simulink model "singlependulum_2"  (R2025a)
settings: Solver=ode15s  StartTime=0.0  StopTime=20  RelTol=1e-3
libraries: fl_lib x32, ee_lib x9, nesl_utility x5
settings Model: Creator=yang  LastModifiedBy=yang

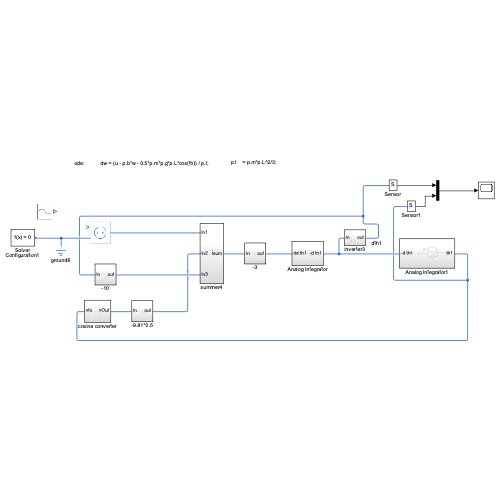
[thumbnail: Simulink's stored preview of the top-level diagram]
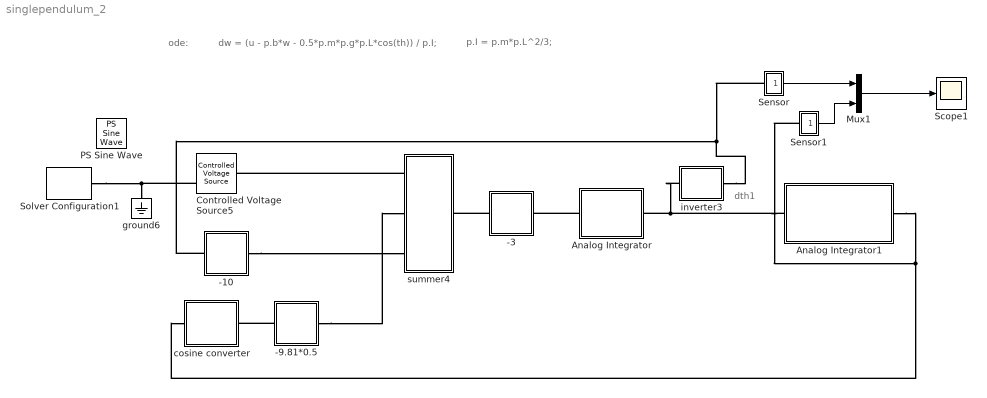
== system singlependulum_2 ==
  note: dth1
  note: ode:
  note: p.I = p.m*p.L^2/3;
  note: dw = (u - p.b*w - 0.5*p.m*p.g*p.L*cos(th)) / p.I;
  -10 : Subsystem
  -3 : Subsystem
  -9.81*0.5 : Subsystem
  Analog Integrator : Subsystem
  Analog Integrator1 : Subsystem
  Controlled Voltage Source5 : fl_lib/Electrical/Electrical Sources/Controlled Voltage Source
  Mux1 : Mux  Inputs=2
  PS Sine Wave : fl_lib/Physical Signals/Sources/PS Sine Wave  amplitude=5  bias=0  frequency_spec=foundation.enum.frequencySpec.angular  frequency_SI=5 Hz  frequency_angular=5 rad/s  phase=0 rad
      settings: InternalSimscapePortConfiguration="{\"Bottom\":[],\"Left\":[],\"Right\":[{\"id\":\"O\",\"label\":\"\",\"type\":\"output\"}],\"Top\":[]}"
  Scope1 : Scope
      settings: ActiveDisplayYMinimum=-2.4953450828768631  ActiveDisplayYMaximum=1.4302884628239119
  Sensor : Subsystem
      mask Display: disp('S')
  Sensor1 : Subsystem
      mask Display: disp('S')
  Solver Configuration1 : nesl_utility/Solver Configuration  PhysicalDomain=network_engine_domain  SubClassName=solver  LeftPortType=input  RightPortType=generic  Tones=[]  Harmonics=[]  SimulateNoise=off  Profile=off  UseLocalSampling=off  EnableSwitchedLinearOptims=on  FrequencyDomain=off  UseCCode=off  RelTol=0.001  AbsTol=1e-06  MinStep=1e-09  ToWorkspace=off  RevertToSquareIcSolve=off  NumHomotopyIterations=100  PhasorMode=off  PhasorModeNumHarmonics=1  ConsistencySolver=NEWTON_XTOL_AFTER_FTOL  IndexReductionMethod=DerivativeReplacement  DoDC=off  ResidualTolerance=1e-09  ConsistencyTolSource=GLOBAL  ConsistencyAbsTol=0.001  ConsistencyRelTol=0.001  ConsistencyTolFactor=0.001  UseLocalSolver=off  LocalSolverChoice=NE_BACKWARD_EULER_ADVANCER  ResolveIndetEquations=on  FunctionEvalNumThread=1  LocalSolverSampleTime=0.001  DoFixedCost=off  MaxNonlinIter=3  MaxModeIter=2  ComputeImpulses=off  ImpulseIterations=2  LinearAlgebra=auto  LinearAlgebraNumThread=0  EquationFormulation=NE_TIME_EF  DelaysMemoryBudget=1024  AutomaticFiltering=on  FilteringTimeConstant=0.001  PartitionStorageMethod=AS_NEEDED  PartitionMemoryBudget=1024  PartitionMethod=ROBUST  MultibodyUseLocalSolver=off  MultibodyLocalSolverChoice=ODE1  MultibodyLocalSolverSampleTime=0.001
  cosine converter : Subsystem
  ground6 : fl_lib/Electrical/Electrical Elements/Electrical Reference
  inverter3 : Subsystem
  summer4 : Subsystem
  wires:
  Sensor/1(Out1) -> Mux1/1
  Sensor1/1(Out1) -> Mux1/2
  Mux1/1 -> Scope1/1
  connections:
  Controlled Voltage Source5/RConn2 -- Solver Configuration1/RConn1 -- ground6/LConn1
  summer4/LConn1 -- Controlled Voltage Source5/LConn1
  Sensor/LConn1 -- -10/LConn1 -- inverter3/RConn1
  Analog Integrator1/RConn1 -- Sensor1/LConn1 -- cosine converter/LConn1
  -9.81*0.5/RConn1 -- summer4/LConn2
  -10/RConn1 -- summer4/LConn3
  -3/LConn1 -- summer4/RConn1
  Analog Integrator/LConn1 -- -3/RConn1
  -9.81*0.5/LConn1 -- cosine converter/RConn1
  Analog Integrator1/LConn1 -- inverter3/LConn1 -- Analog Integrator/RConn1

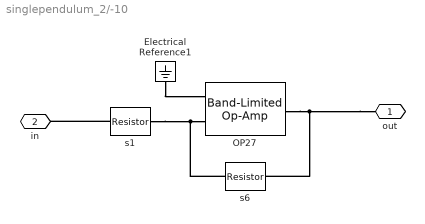
== system singlependulum_2/-10 ==
  Electrical Reference1 : fl_lib/Electrical/Electrical Elements/Electrical Reference
  OP27 : ee_lib/Integrated Circuits/Band-Limited Op-Amp  A=1.8E6  Rin=4e6 Ohm  Rout=70 Ohm  Vmin=-24 V  Vmax=24 V  Vdotmax=2.8E6 V/s  f=8E6 Hz  V0=0 V
  s1 : fl_lib/Electrical/Electrical Elements/Resistor  R=1E3 Ohm  i_specify=off  i_priority=None  i=0 A  i_nominal_specify=off  i_nominal_value=1  i_nominal_unit=A  v_specify=off  v_priority=None  v=0 V  v_nominal_specify=off  v_nominal_value=1  v_nominal_unit=V
  s6 : fl_lib/Electrical/Electrical Elements/Resistor  R=10E3 Ohm  i_specify=off  i_priority=None  i=0 A  i_nominal_specify=off  i_nominal_value=1  i_nominal_unit=A  v_specify=off  v_priority=None  v=0 V  v_nominal_specify=off  v_nominal_value=1  v_nominal_unit=V
  out : PMIOPort  Side=Right
  in : PMIOPort  Port=2  Side=Left
  connections:
  OP27/LConn2 -- s1/RConn1 -- s6/LConn1
  s1/LConn1 -- in/RConn1
  Electrical Reference1/LConn1 -- OP27/LConn1
  out/RConn1 -- s6/RConn1 -- OP27/RConn1

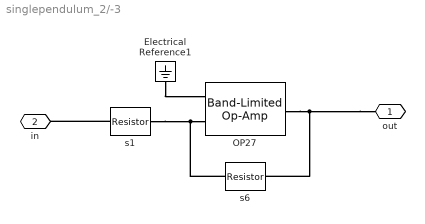
== system singlependulum_2/-3 ==
  Electrical Reference1 : fl_lib/Electrical/Electrical Elements/Electrical Reference
  OP27 : ee_lib/Integrated Circuits/Band-Limited Op-Amp  A=1.8E6  Rin=4e6 Ohm  Rout=70 Ohm  Vmin=-24 V  Vmax=24 V  Vdotmax=2.8E6 V/s  f=8E6 Hz  V0=0 V
  s1 : fl_lib/Electrical/Electrical Elements/Resistor  R=1E3 Ohm  i_specify=off  i_priority=None  i=0 A  i_nominal_specify=off  i_nominal_value=1  i_nominal_unit=A  v_specify=off  v_priority=None  v=0 V  v_nominal_specify=off  v_nominal_value=1  v_nominal_unit=V
  s6 : fl_lib/Electrical/Electrical Elements/Resistor  R=3E3 Ohm  i_specify=off  i_priority=None  i=0 A  i_nominal_specify=off  i_nominal_value=1  i_nominal_unit=A  v_specify=off  v_priority=None  v=0 V  v_nominal_specify=off  v_nominal_value=1  v_nominal_unit=V
  out : PMIOPort  Side=Right
  in : PMIOPort  Port=2  Side=Left
  connections:
  OP27/LConn2 -- s1/RConn1 -- s6/LConn1
  s1/LConn1 -- in/RConn1
  Electrical Reference1/LConn1 -- OP27/LConn1
  out/RConn1 -- s6/RConn1 -- OP27/RConn1

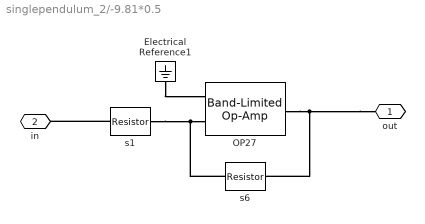
== system singlependulum_2/-9.81*0.5 ==
  Electrical Reference1 : fl_lib/Electrical/Electrical Elements/Electrical Reference
  OP27 : ee_lib/Integrated Circuits/Band-Limited Op-Amp  A=1.8E6  Rin=4e6 Ohm  Rout=70 Ohm  Vmin=-24 V  Vmax=24 V  Vdotmax=2.8E6 V/s  f=8E6 Hz  V0=0 V
  s1 : fl_lib/Electrical/Electrical Elements/Resistor  R=1E3 Ohm  i_specify=off  i_priority=None  i=0 A  i_nominal_specify=off  i_nominal_value=1  i_nominal_unit=A  v_specify=off  v_priority=None  v=0 V  v_nominal_specify=off  v_nominal_value=1  v_nominal_unit=V
  s6 : fl_lib/Electrical/Electrical Elements/Resistor  R=9.81*0.5E3 Ohm  i_specify=off  i_priority=None  i=0 A  i_nominal_specify=off  i_nominal_value=1  i_nominal_unit=A  v_specify=off  v_priority=None  v=0 V  v_nominal_specify=off  v_nominal_value=1  v_nominal_unit=V
  out : PMIOPort  Side=Right
  in : PMIOPort  Port=2  Side=Left
  connections:
  OP27/LConn2 -- s1/RConn1 -- s6/LConn1
  s1/LConn1 -- in/RConn1
  Electrical Reference1/LConn1 -- OP27/LConn1
  out/RConn1 -- s6/RConn1 -- OP27/RConn1

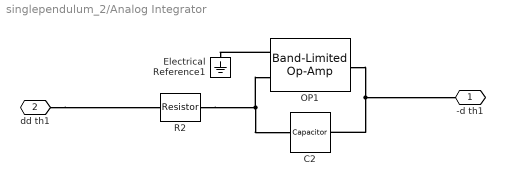
== system singlependulum_2/Analog Integrator ==
  C2 : ee_lib/Passive/Capacitor  cap_option=ee.enum.passive.capacitor.capOption.const  c=1e-9 F  Cvec=[1e-05, 1e-06] F  Vvec=[0, 10] V  CV_table_symmetry=ee.enum.passive.capacitor.tableSymmetry.yes  f_vec=[1, 10] kHz  DFext_vec=[.8, 1.2]  enable_C_tol=ee.enum.toleranceApplication.none  averaging_period=0 s  C_tol=5  tol_distribution=ee.enum.toleranceDistribution.uniform  nSigma=4  r=1e-6 Ohm  g=0 1/Ohm  enable_operating_limits=ee.enum.enable.no  operating_limit_action=ee.enum.passive.reportOpLim.warn  max_working_voltage_range=[-25, 25] V  power_rating=1 W  maxTemperature=85 degC  thermalEnable=false  thermalMass=1 J/K  i_specify=off  i_priority=None  i=0 A  i_nominal_specify=off  i_nominal_value=1  i_nominal_unit=A  v_specify=off  v_priority=High  v=1 V  v_nominal_specify=off  v_nominal_value=1  v_nominal_unit=V  vc_specify=on  vc_priority=High  vc=0 V  vc_nominal_specify=off  vc_nominal_value=1  vc_nominal_unit=V  T_specify=off  T_priority=None  T=298.15 K  T_nominal_specify=off  T_nominal_value=1  T_nominal_unit=K
  Electrical Reference1 : fl_lib/Electrical/Electrical Elements/Electrical Reference
  OP1 : ee_lib/Integrated Circuits/Band-Limited Op-Amp  A=1.8E6  Rin=4e6 Ohm  Rout=70 Ohm  Vmin=-10 V  Vmax=10 V  Vdotmax=2.8E6 V/s  f=8E6 Hz  V0=0 V
  R2 : fl_lib/Electrical/Electrical Elements/Resistor  R=(1E9)/1 Ohm  i_specify=off  i_priority=None  i=0 A  i_nominal_specify=off  i_nominal_value=1  i_nominal_unit=A  v_specify=off  v_priority=None  v=0 V  v_nominal_specify=off  v_nominal_value=1  v_nominal_unit=V
  -d th1 : PMIOPort  Side=Right
  dd th1 : PMIOPort  Port=2  Side=Left
  connections:
  OP1/LConn1 -- Electrical Reference1/LConn1
  R2/RConn1 -- OP1/LConn2 -- C2/LConn1
  C2/RConn1 -- -d th1/RConn1 -- OP1/RConn1
  dd th1/RConn1 -- R2/LConn1

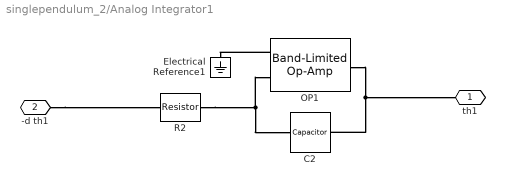
== system singlependulum_2/Analog Integrator1 ==
  C2 : ee_lib/Passive/Capacitor  cap_option=ee.enum.passive.capacitor.capOption.const  c=1e-9 F  Cvec=[1e-05, 1e-06] F  Vvec=[0, 10] V  CV_table_symmetry=ee.enum.passive.capacitor.tableSymmetry.yes  f_vec=[1, 10] kHz  DFext_vec=[.8, 1.2]  enable_C_tol=ee.enum.toleranceApplication.none  averaging_period=0 s  C_tol=5  tol_distribution=ee.enum.toleranceDistribution.uniform  nSigma=4  r=1e-6 Ohm  g=0 1/Ohm  enable_operating_limits=ee.enum.enable.no  operating_limit_action=ee.enum.passive.reportOpLim.warn  max_working_voltage_range=[-25, 25] V  power_rating=1 W  maxTemperature=85 degC  thermalEnable=false  thermalMass=1 J/K  i_specify=off  i_priority=None  i=0 A  i_nominal_specify=off  i_nominal_value=1  i_nominal_unit=A  v_specify=off  v_priority=High  v=1 V  v_nominal_specify=off  v_nominal_value=1  v_nominal_unit=V  vc_specify=on  vc_priority=High  vc=0 V  vc_nominal_specify=off  vc_nominal_value=1  vc_nominal_unit=V  T_specify=off  T_priority=None  T=298.15 K  T_nominal_specify=off  T_nominal_value=1  T_nominal_unit=K
  Electrical Reference1 : fl_lib/Electrical/Electrical Elements/Electrical Reference
  OP1 : ee_lib/Integrated Circuits/Band-Limited Op-Amp  A=1.8E6  Rin=4e6 Ohm  Rout=70 Ohm  Vmin=-10 V  Vmax=10 V  Vdotmax=2.8E6 V/s  f=8E6 Hz  V0=0 V
  R2 : fl_lib/Electrical/Electrical Elements/Resistor  R=(1E9)/1 Ohm  i_specify=off  i_priority=None  i=0 A  i_nominal_specify=off  i_nominal_value=1  i_nominal_unit=A  v_specify=off  v_priority=None  v=0 V  v_nominal_specify=off  v_nominal_value=1  v_nominal_unit=V
  th1 : PMIOPort  Side=Right
  -d th1 : PMIOPort  Port=2  Side=Left
  connections:
  OP1/LConn1 -- Electrical Reference1/LConn1
  R2/RConn1 -- OP1/LConn2 -- C2/LConn1
  C2/RConn1 -- th1/RConn1 -- OP1/RConn1
  -d th1/RConn1 -- R2/LConn1

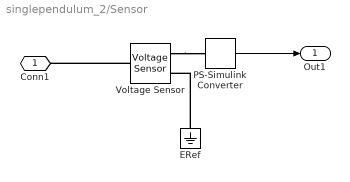
== system singlependulum_2/Sensor ==
  ERef : fl_lib/Electrical/Electrical Elements/Electrical Reference
  PS-Simulink Converter : nesl_utility/PS-Simulink Converter  PhysicalDomain=network_engine_domain  SubClassName=ps_output  LeftPortType=input  RightPortType=output  PseudoPeriodic=off  Frequencies=[]  VectorFormat=1-D array  Unit=1  AffineConversion=off
  Voltage Sensor : fl_lib/Electrical/Electrical Sensors/Voltage Sensor
  Conn1 : PMIOPort  Side=Left
  Out1 : Outport  VectorParamsAs1DForOutWhenUnconnected=off
  wires:
  PS-Simulink Converter/1 -> Out1/1
  connections:
  ERef/LConn1 -- Voltage Sensor/RConn2
  Voltage Sensor/RConn1 -- PS-Simulink Converter/LConn1
  Voltage Sensor/LConn1 -- Conn1/RConn1

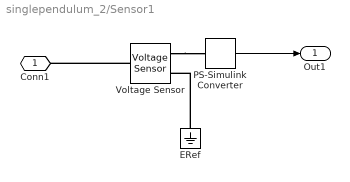
== system singlependulum_2/Sensor1 ==
  ERef : fl_lib/Electrical/Electrical Elements/Electrical Reference
  PS-Simulink Converter : nesl_utility/PS-Simulink Converter  PhysicalDomain=network_engine_domain  SubClassName=ps_output  LeftPortType=input  RightPortType=output  PseudoPeriodic=off  Frequencies=[]  VectorFormat=1-D array  Unit=1  AffineConversion=off
  Voltage Sensor : fl_lib/Electrical/Electrical Sensors/Voltage Sensor
  Conn1 : PMIOPort  Side=Left
  Out1 : Outport  VectorParamsAs1DForOutWhenUnconnected=off
  wires:
  PS-Simulink Converter/1 -> Out1/1
  connections:
  ERef/LConn1 -- Voltage Sensor/RConn2
  Voltage Sensor/RConn1 -- PS-Simulink Converter/LConn1
  Voltage Sensor/LConn1 -- Conn1/RConn1

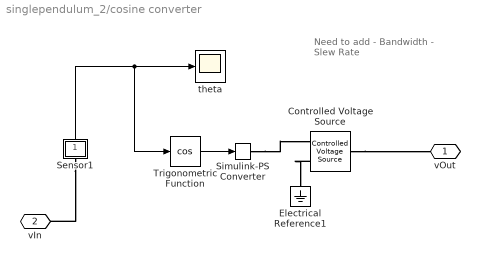
== system singlependulum_2/cosine converter ==
  note: Need to add
      | - Bandwidth
      | - Slew Rate
  Controlled Voltage Source : fl_lib/Electrical/Electrical Sources/Controlled Voltage Source
  Electrical Reference1 : fl_lib/Electrical/Electrical Elements/Electrical Reference
  Sensor1 : Subsystem
      mask Display: disp('S')
  Simulink-PS Converter : nesl_utility/Simulink-PS Converter  PhysicalDomain=network_engine_domain  SubClassName=ps_input  LeftPortType=input  RightPortType=output  PseudoPeriodic=off  Frequencies=[]  NoiseDistribution=none  NoiseParameters=[]  Unit=1  AffineConversion=off  FilteringAndDerivatives=provide  SimscapeFilterOrder=1  InputFilterTimeConstant=0.001  UdotUserProvided=0
  Trigonometric Function : Trigonometry  Operator=cos
  theta : Scope
      settings: ActiveDisplayYMinimum=-0.15074  ActiveDisplayYMaximum=0.77598  DataLoggingVariableName=ScopeData2
  vOut : PMIOPort  Side=Right
  vIn : PMIOPort  Port=2  Side=Left
  wires:
  Sensor1/1(Out1) -> theta/1, Trigonometric Function/1
  Trigonometric Function/1 -> Simulink-PS Converter/1
  connections:
  Controlled Voltage Source/RConn2 -- Electrical Reference1/LConn1
  Simulink-PS Converter/RConn1 -- Controlled Voltage Source/RConn1
  Sensor1/LConn1 -- vIn/RConn1
  Controlled Voltage Source/LConn1 -- vOut/RConn1

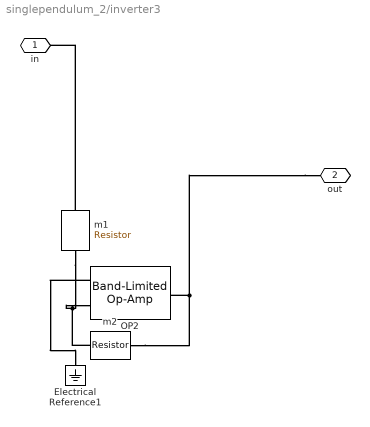
== system singlependulum_2/inverter3 ==
  Electrical Reference1 : fl_lib/Electrical/Electrical Elements/Electrical Reference
  OP2 : ee_lib/Integrated Circuits/Band-Limited Op-Amp  A=1.8E6  Rin=4e6 Ohm  Rout=70 Ohm  Vmin=-10 V  Vmax=10 V  Vdotmax=2.8E6 V/s  f=8E6 Hz  V0=0 V
  m1 : fl_lib/Electrical/Electrical Elements/Resistor  R=1E3 Ohm  i_specify=off  i_priority=None  i=0 A  i_nominal_specify=off  i_nominal_value=1  i_nominal_unit=A  v_specify=off  v_priority=None  v=0 V  v_nominal_specify=off  v_nominal_value=1  v_nominal_unit=V
  m2 : fl_lib/Electrical/Electrical Elements/Resistor  R=1E3 Ohm  i_specify=off  i_priority=None  i=0 A  i_nominal_specify=off  i_nominal_value=1  i_nominal_unit=A  v_specify=off  v_priority=None  v=0 V  v_nominal_specify=off  v_nominal_value=1  v_nominal_unit=V
  in : PMIOPort  Side=Left
  out : PMIOPort  Port=2  Side=Right
  connections:
  m1/LConn1 -- in/RConn1
  out/RConn1 -- OP2/RConn1 -- m2/LConn1
  OP2/LConn2 -- m1/RConn1 -- m2/RConn1
  OP2/LConn1 -- Electrical Reference1/LConn1

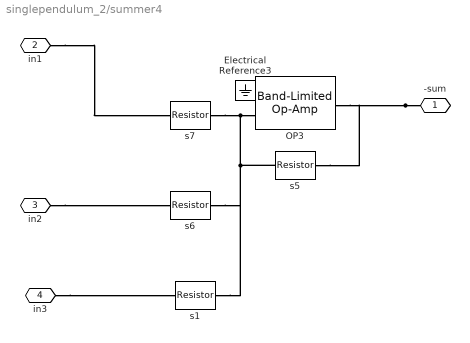
== system singlependulum_2/summer4 ==
  Electrical Reference3 : fl_lib/Electrical/Electrical Elements/Electrical Reference
  OP3 : ee_lib/Integrated Circuits/Band-Limited Op-Amp  A=1.8E6  Rin=4e6 Ohm  Rout=70 Ohm  Vmin=-10 V  Vmax=10 V  Vdotmax=2.8E6 V/s  f=8E6 Hz  V0=0 V
  s{1,5..7} (4 alike) : fl_lib/Electrical/Electrical Elements/Resistor  R=10E3 Ohm  i_specify=off  i_priority=None  i=0 A  i_nominal_specify=off  i_nominal_value=1  i_nominal_unit=A  v_specify=off  v_priority=None  v=0 V  v_nominal_specify=off  v_nominal_value=1  v_nominal_unit=V
  -sum : PMIOPort  Side=Right
  in1 : PMIOPort  Port=2  Side=Left
  in2 : PMIOPort  Port=3  Side=Left
  in3 : PMIOPort  Port=4  Side=Left
  connections:
  in3/RConn1 -- s1/LConn1
  in1/RConn1 -- s7/LConn1
  in2/RConn1 -- s6/LConn1
  Electrical Reference3/LConn1 -- OP3/LConn1
  -sum/RConn1 -- s5/RConn1 -- OP3/RConn1
  OP3/LConn2 -- s7/RConn1 -- s1/RConn1 -- s6/RConn1 -- s5/LConn1

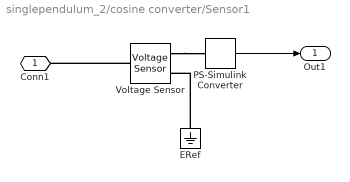
== system singlependulum_2/cosine converter/Sensor1 ==
  ERef : fl_lib/Electrical/Electrical Elements/Electrical Reference
  PS-Simulink Converter : nesl_utility/PS-Simulink Converter  PhysicalDomain=network_engine_domain  SubClassName=ps_output  LeftPortType=input  RightPortType=output  PseudoPeriodic=off  Frequencies=[]  VectorFormat=1-D array  Unit=1  AffineConversion=off
  Voltage Sensor : fl_lib/Electrical/Electrical Sensors/Voltage Sensor
  Conn1 : PMIOPort  Side=Left
  Out1 : Outport  VectorParamsAs1DForOutWhenUnconnected=off
  wires:
  PS-Simulink Converter/1 -> Out1/1
  connections:
  ERef/LConn1 -- Voltage Sensor/RConn2
  Voltage Sensor/RConn1 -- PS-Simulink Converter/LConn1
  Voltage Sensor/LConn1 -- Conn1/RConn1
